simulink model "VLPF"  (R2020b)
settings: Solver=VariableStepAuto  StartTime=0.0  StopTime=20  RelTol=1e-3
libraries: cstblocks x2
settings Model: Creator=racarla1  LastModifiedBy=racarla1

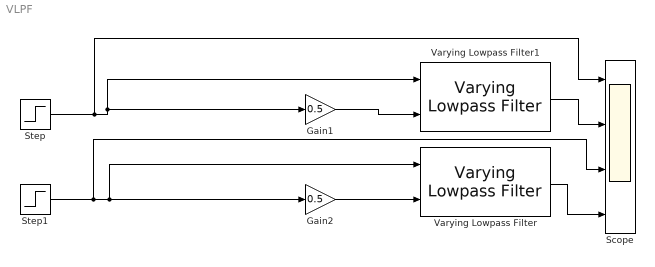
== system VLPF ==
  Gain1 : Gain  Gain=0.5
  Gain2 : Gain  Gain=0.5
  Scope : Scope  NumInputPorts=4
  Step : Step  SampleTime=0.01
  Step1 : Step  After=5  SampleTime=0.01
  Varying Lowpass Filter : cstblocks/Linear Parameter Varying/Varying Lowpass Filter  N=1
  Varying Lowpass Filter1 : cstblocks/Linear Parameter Varying/Varying Lowpass Filter  N=1
  wires:
  Varying Lowpass Filter/1 -> Scope/4
  Step/1 -> Gain1/1, Varying Lowpass Filter1/1, Scope/1
  Gain2/1 -> Varying Lowpass Filter/2
  Varying Lowpass Filter1/1 -> Scope/2
  Gain1/1 -> Varying Lowpass Filter1/2
  Step1/1 -> Gain2/1, Varying Lowpass Filter/1, Scope/3
